simulink model "potential_field_controller"  (R2020b)
settings: Solver=VariableStepAuto  StartTime=0.0  StopTime=inf  RelTol=1e-3
values from neighbouring files (symbols this model uses):
  nObst = size(obstacles,2)    [setupPFC.m]
  obstacles = getObstaclepoints()    [setupPFC.m]
  timeDelay = FMS.Ts*4    [setupPFC.m]
  waypoints = getWaypoints()    [setupPFC.m]
undefined symbols (not defined in the file or in its folder): ssH, ssPitch, ssPitch2U, ssRoll, ssRoll2V, ssYaw
libraries: simulink x2, ARBlocks x1
settings Model: Creator=Adarsh  LastModifiedBy=Adarsh

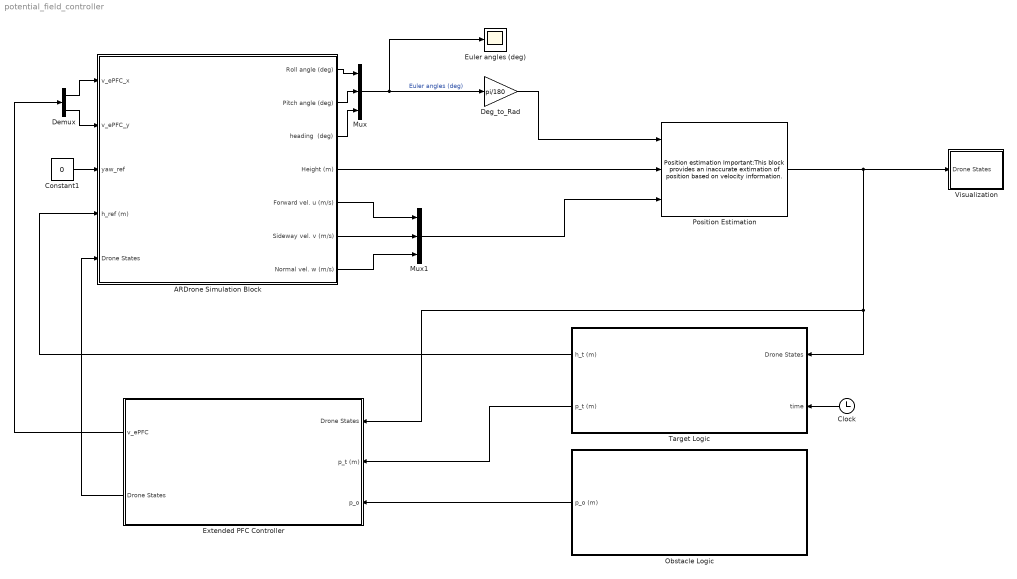
== system potential_field_controller ==
  ARDrone Simulation Block : Subsystem  AncestorBlock=ARBlocks/ARDrone Simulation Block
  Clock : Clock
  Constant1 : Constant  Value=0
  Deg_to_Rad : Gain  Gain=pi/180
  Demux : Demux  Outputs=2
  Euler angles (deg) : Scope
  Extended PFC Controller : Subsystem  AncestorBlock=ARBlocks/Baseline Controller
  Mux : Mux  Inputs=3
  Mux1 : Mux  Inputs=3
  Obstacle Logic : Subsystem  AncestorBlock=ARBlocks/Guidance logic
  "Position Estimation " : ARBlocks/Position estimation Important:This block provides an  inaccurate extimation of position  based on  velocity information.   SystemSampleTime=-1  VariantActivationTime=update diagram  Latency=0  AutoFrameSizeCalculation=off
  Target Logic : Subsystem  AncestorBlock=ARBlocks/Guidance logic
  Visualization : Subsystem
  wires:
  ARDrone Simulation Block/1(Roll angle (deg)) -> Mux/1
  ARDrone Simulation Block/2(Pitch angle (deg)) -> Mux/2
  ARDrone Simulation Block/3(heading  (deg)) -> Mux/3
  Deg_to_Rad/1 -> "Position Estimation "/1
  ARDrone Simulation Block/4(Height (m)) -> "Position Estimation "/2
  ARDrone Simulation Block/5(Forward vel. u (m/s)) -> Mux1/1
  ARDrone Simulation Block/6(Sideway vel. v (m/s)) -> Mux1/2
  ARDrone Simulation Block/7(Normal vel. w (m/s)) -> Mux1/3
  Mux1/1 -> "Position Estimation "/3
  "Position Estimation "/1 -> Visualization/1(Drone States), Target Logic/1(Drone States), Extended PFC Controller/1("Drone States ")
  Obstacle Logic/1(p_o (m)) -> Extended PFC Controller/3(p_o)
  Target Logic/2(p_t (m)) -> Extended PFC Controller/2(p_t (m))
  Target Logic/1(h_t (m)) -> ARDrone Simulation Block/4(h_ref (m))
  Clock/1 -> Target Logic/2(time)
  Mux/1 -> Euler angles (deg)/1, Deg_to_Rad/1  "Euler angles (deg)"
  Demux/1 -> ARDrone Simulation Block/1(v_ePFC_x)
  Demux/2 -> ARDrone Simulation Block/2(v_ePFC_y)
  Extended PFC Controller/1(v_ePFC) -> Demux/1
  Constant1/1 -> ARDrone Simulation Block/3(yaw_ref)
  Extended PFC Controller/2(Drone States) -> ARDrone Simulation Block/5(Drone States)

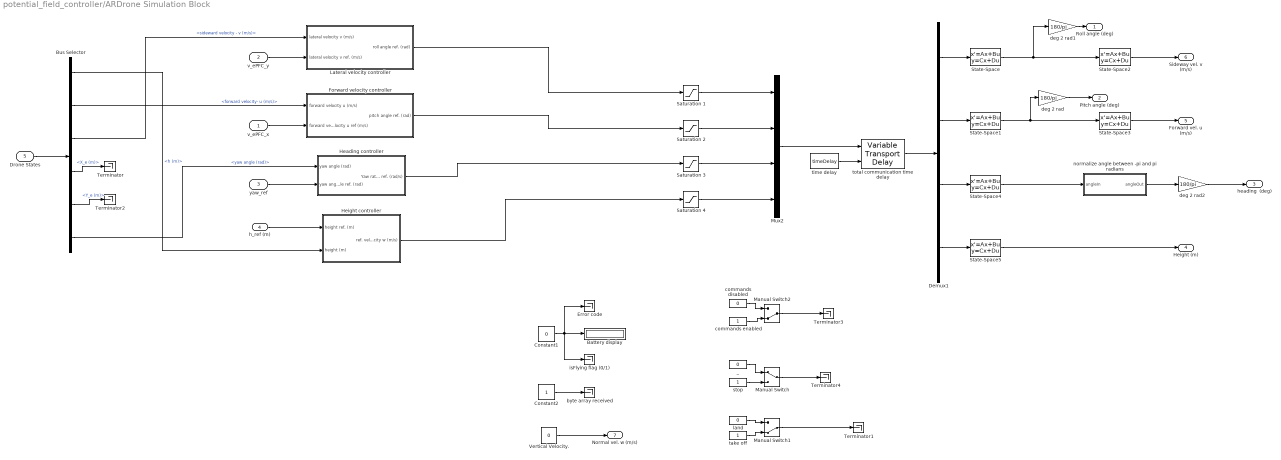
== system potential_field_controller/ARDrone Simulation Block ==
  v_ePFC_x : Inport
  v_ePFC_y : Inport  Port=2
  yaw_ref : Inport  Port=3
  h_ref (m) : Inport  Port=4
  Drone States : Inport  Port=5
  Battery display : Display
  Bus Selector : BusSelector  OutputSignals=h (m),forward velocity- u (m/s),sideward velocity - v (m/s),X_e (m),Y_e (m),yaw angle (rad)
  Constant1 : Constant  Value=0
  Constant2 : Constant
  Demux1 : Demux
  Error code : Terminator
  "Forward velocity controller " : Subsystem
  Heading controller : Subsystem
  "Height controller " : Subsystem
  Lateral velocity controller : Subsystem
  Manual Switch : ManualSwitch
  Manual Switch1 : ManualSwitch  CurrentSetting=0
  Manual Switch2 : ManualSwitch  CurrentSetting=0
  Mux2 : Mux
  Saturation {1..4} (4 alike) : Saturate  UpperLimit=1  LowerLimit=-1
  State-Space : StateSpace  A=ssRoll.a  B=ssRoll.b  C=ssRoll.c  D=ssRoll.d  InitialCondition=0
  State-Space1 : StateSpace  A=ssPitch.a  B=ssPitch.b  C=ssPitch.c  D=ssPitch.d  InitialCondition=0
  State-Space2 : StateSpace  A=ssRoll2V.a  B=ssRoll2V.b  C=ssRoll2V.c  D=ssRoll2V.d  InitialCondition=0
  State-Space3 : StateSpace  A=ssPitch2U.a  B=ssPitch2U.b  C=ssPitch2U.c  D=ssPitch2U.d  InitialCondition=0
  State-Space4 : StateSpace  A=ssYaw.a  B=ssYaw.b  C=ssYaw.c  D=ssYaw.d  InitialCondition=0
  State-Space5 : StateSpace  A=ssH.a  B=ssH.b  C=ssH.c  D=ssH.d  InitialCondition=0
  Terminator{,1..4} (5 alike) : Terminator
  "Vertical Velocity. " : Constant  Value=0
  _ : Constant  Value=0
  byte array received : Terminator
  commands disabled : Constant  Value=0
  commands enabled : Constant
  deg 2 rad : Gain  Gain=180/pi
  deg 2 rad1 : Gain  Gain=180/pi
  deg 2 rad2 : Gain  Gain=180/pi
  isFlying flag (0/1) : Terminator
  land : Constant  Value=0
  normalize angle between -pi and pi radians : MATLAB Function  TreatAsAtomicUnit=on
  stop : Constant
  take off : Constant
  time delay : Constant  Value=timeDelay
  total communication time delay : VariableTransportDelay  MaximumDelay=10  InitialOutput=[0 0 0 0]  MaximumPoints=4096
  Roll angle (deg) : Outport
  Pitch angle (deg) : Outport  Port=2
  heading  (deg) : Outport  Port=3
  Height (m) : Outport  Port=4
  Forward vel. u (m/s) : Outport  Port=5
  Sideway vel. v (m/s) : Outport  Port=6
  Normal vel. w (m/s) : Outport  Port=7
  wires:
  "Vertical Velocity. "/1 -> Normal vel. w (m/s)/1
  deg 2 rad2/1 -> heading  (deg)/1
  deg 2 rad1/1 -> Roll angle (deg)/1
  deg 2 rad/1 -> Pitch angle (deg)/1
  normalize angle between -pi and pi radians/1(angleOut) -> deg 2 rad2/1
  State-Space5/1 -> Height (m)/1
  State-Space3/1 -> Forward vel. u (m/s)/1
  State-Space2/1 -> Sideway vel. v (m/s)/1
  State-Space4/1 -> normalize angle between -pi and pi radians/1(angleIn)
  Demux1/3 -> State-Space4/1
  Demux1/2 -> State-Space1/1
  Saturation 4/1 -> Mux2/4
  Saturation 3/1 -> Mux2/3
  Saturation 2/1 -> Mux2/2
  Saturation 1/1 -> Mux2/1
  total communication time delay/1 -> Demux1/1
  Mux2/1 -> total communication time delay/1
  time delay/1 -> total communication time delay/2
  State-Space1/1 -> State-Space3/1, deg 2 rad/1
  State-Space/1 -> State-Space2/1, deg 2 rad1/1
  Demux1/4 -> State-Space5/1
  Demux1/1 -> State-Space/1
  "Height controller "/1(ref. velocity w (m/s)) -> Saturation 4/1
  "Forward velocity controller "/1(pitch angle ref. (rad)) -> Saturation 2/1
  Lateral velocity controller/1(roll angle ref. (rad)) -> Saturation 1/1
  land/1 -> Manual Switch1/1
  Manual Switch1/1 -> Terminator1/1
  take off/1 -> Manual Switch1/2
  commands disabled/1 -> Manual Switch2/1
  commands enabled/1 -> Manual Switch2/2
  Manual Switch2/1 -> Terminator3/1
  Manual Switch/1 -> Terminator4/1
  stop/1 -> Manual Switch/2
  _/1 -> Manual Switch/1
  Constant1/1 -> Battery display/1, Error code/1, isFlying flag (0/1)/1
  Constant2/1 -> byte array received/1
  yaw_ref/1 -> Heading controller/2(yaw angle ref. (rad))
  Heading controller/1(Yaw rate ref. (rad/s)) -> Saturation 3/1
  v_ePFC_y/1 -> Lateral velocity controller/2(lateral velocity v ref. (m/s))
  v_ePFC_x/1 -> "Forward velocity controller "/2(forward velocity u ref (m/s))
  h_ref (m)/1 -> "Height controller "/1(height ref. (m))
  Drone States/1 -> Bus Selector/1
  Bus Selector/1 -> "Height controller "/2(height (m))  "<h (m)>"
  Bus Selector/2 -> "Forward velocity controller "/1(forward velocity u (m/s))  "<forward velocity- u (m/s)>"
  Bus Selector/3 -> Lateral velocity controller/1(lateral velocity v (m/s))  "<sideward velocity - v (m/s)>"
  Bus Selector/6 -> Heading controller/1(yaw angle (rad))  "<yaw angle (rad)>"
  Bus Selector/4 -> Terminator/1  "<X_e (m)>"
  Bus Selector/5 -> Terminator2/1  "<Y_e (m)>"

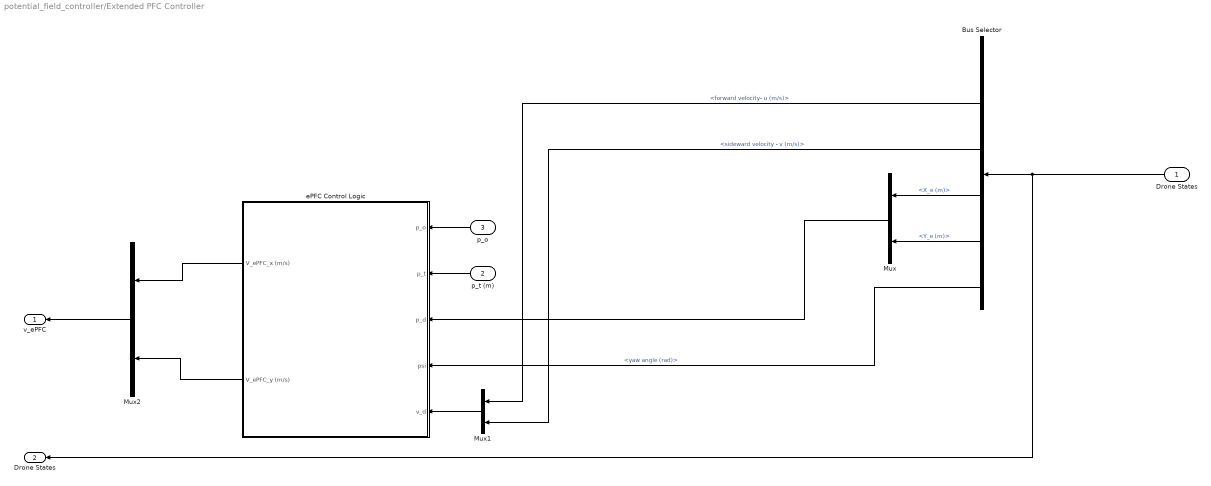
== system potential_field_controller/Extended PFC Controller ==
  "Drone States " : Inport
  p_t (m) : Inport  Port=2
  p_o : Inport  Port=3
  Bus Selector : BusSelector  OutputSignals=h (m),forward velocity- u (m/s),sideward velocity - v (m/s),X_e (m),Y_e (m),yaw angle (rad)
  Mux : Mux  Inputs=2
  Mux1 : Mux  Inputs=2
  Mux2 : Mux  Inputs=2
  ePFC Control Logic : Subsystem
  v_ePFC : Outport
  Drone States : Outport  Port=2
  wires:
  Bus Selector/6 -> ePFC Control Logic/4(psi)  "<yaw angle (rad)>"
  Bus Selector/2 -> Mux1/1  "<forward velocity- u (m/s)>"
  p_t (m)/1 -> ePFC Control Logic/2(p_t)
  Bus Selector/3 -> Mux1/2  "<sideward velocity - v (m/s)>"
  p_o/1 -> ePFC Control Logic/1(p_o)
  Bus Selector/4 -> Mux/1  "<X_e (m)>"
  Bus Selector/5 -> Mux/2  "<Y_e (m)>"
  Mux/1 -> ePFC Control Logic/3(p_d)
  Mux1/1 -> ePFC Control Logic/5(v_d)
  "Drone States "/1 -> Drone States/1, Bus Selector/1
  ePFC Control Logic/2(V_ePFC_y (m/s)) -> Mux2/2
  ePFC Control Logic/1(V_ePFC_x (m/s)) -> Mux2/1
  Mux2/1 -> v_ePFC/1

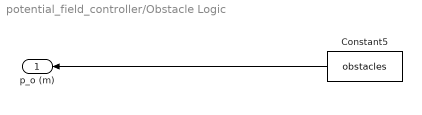
== system potential_field_controller/Obstacle Logic ==
  Constant5 : Constant  Value=obstacles  VectorParams1D=off
  p_o (m) : Outport
  wires:
  Constant5/1 -> p_o (m)/1

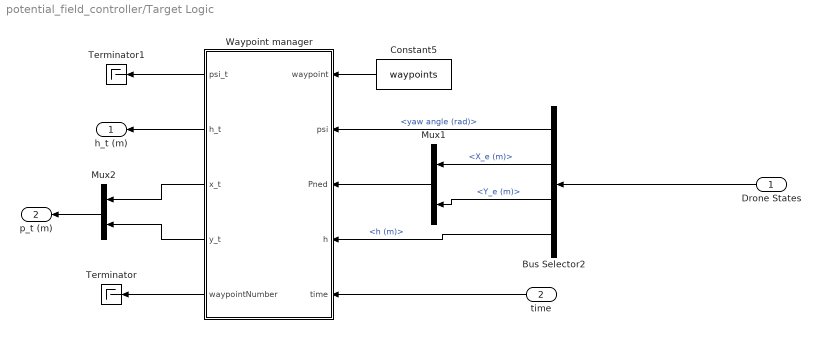
== system potential_field_controller/Target Logic ==
  Drone States : Inport
  time : Inport  Port=2
  Bus Selector2 : BusSelector  OutputSignals=yaw angle (rad),X_e (m),Y_e (m),h (m)
  Constant5 : Constant  Value=waypoints  VectorParams1D=off
  Mux1 : Mux  Inputs=2
  Mux2 : Mux  Inputs=2
  Terminator : Terminator
  Terminator1 : Terminator
  "Waypoint manager " : MATLAB Function  TreatAsAtomicUnit=on
  h_t (m) : Outport
  p_t (m) : Outport  Port=2
  wires:
  Constant5/1 -> "Waypoint manager "/1(waypoint)
  "Waypoint manager "/1(psi_t) -> Terminator1/1
  "Waypoint manager "/5(waypointNumber) -> Terminator/1
  Bus Selector2/4 -> "Waypoint manager "/4(h)  "<h (m)>"
  "Waypoint manager "/4(y_t) -> Mux2/2
  "Waypoint manager "/3(x_t) -> Mux2/1
  "Waypoint manager "/2(h_t) -> h_t (m)/1
  Mux1/1 -> "Waypoint manager "/3(Pned)
  Bus Selector2/1 -> "Waypoint manager "/2(psi)  "<yaw angle (rad)>"
  Bus Selector2/3 -> Mux1/2  "<Y_e (m)>"
  Bus Selector2/2 -> Mux1/1  "<X_e (m)>"
  Mux2/1 -> p_t (m)/1
  Drone States/1 -> Bus Selector2/1
  time/1 -> "Waypoint manager "/5(time)

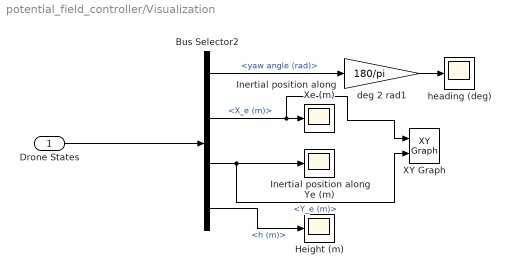
== system potential_field_controller/Visualization ==
  Drone States : Inport
  Bus Selector2 : BusSelector  OutputSignals=yaw angle (rad),X_e (m),Y_e (m),h (m)
  Height (m) : Scope
  Inertial position along Xe (m) : Scope
  Inertial position along Ye (m) : Scope
  XY Graph : simulink/Sinks/XY Graph  xmin=-3  xmax=3  ymin=-2  ymax=2  st=-1
  deg 2 rad1 : Gain  Gain=180/pi
  heading (deg) : Scope
  wires:
  Drone States/1 -> Bus Selector2/1
  Bus Selector2/1 -> deg 2 rad1/1  "<yaw angle (rad)>"
  Bus Selector2/2 -> XY Graph/1, Inertial position along Xe (m)/1  "<X_e (m)>"
  Bus Selector2/3 -> Inertial position along Ye (m)/1, XY Graph/2  "<Y_e (m)>"
  Bus Selector2/4 -> Height (m)/1  "<h (m)>"
  deg 2 rad1/1 -> heading (deg)/1

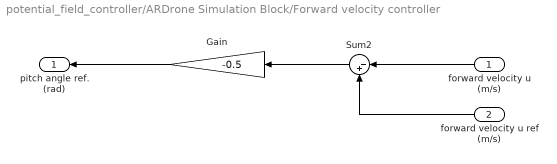
== system potential_field_controller/ARDrone Simulation Block/Forward velocity controller  ==
  forward velocity u (m/s) : Inport
  forward velocity u ref (m/s) : Inport  Port=2
  Gain : Gain  Gain=-0.5
  Sum2 : Sum  Inputs=|-+
  pitch angle ref. (rad) : Outport
  wires:
  forward velocity u (m/s)/1 -> Sum2/1
  Sum2/1 -> Gain/1
  Gain/1 -> pitch angle ref. (rad)/1
  forward velocity u ref (m/s)/1 -> Sum2/2

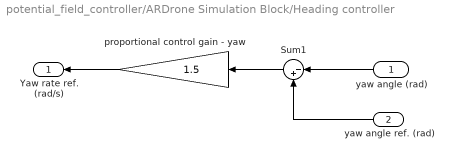
== system potential_field_controller/ARDrone Simulation Block/Heading controller ==
  yaw angle (rad) : Inport
  yaw angle ref. (rad) : Inport  Port=2
  Sum1 : Sum  Inputs=|-+
  proportional control gain - yaw : Gain  Gain=1.5
  Yaw rate ref. (rad/s) : Outport
  wires:
  yaw angle (rad)/1 -> Sum1/1
  proportional control gain - yaw/1 -> Yaw rate ref. (rad/s)/1
  Sum1/1 -> proportional control gain - yaw/1
  yaw angle ref. (rad)/1 -> Sum1/2

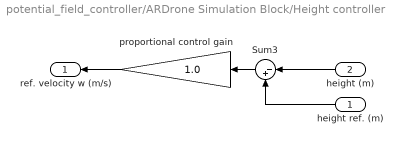
== system potential_field_controller/ARDrone Simulation Block/Height controller  ==
  height ref. (m) : Inport
  height (m) : Inport  Port=2
  Sum3 : Sum  Inputs=|-+
  proportional control gain : Gain  Gain=1.0
  ref. velocity w (m/s) : Outport
  wires:
  proportional control gain/1 -> ref. velocity w (m/s)/1
  Sum3/1 -> proportional control gain/1
  height (m)/1 -> Sum3/1
  height ref. (m)/1 -> Sum3/2

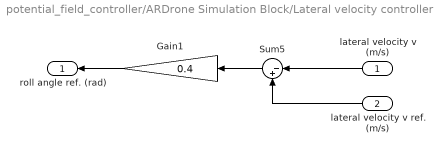
== system potential_field_controller/ARDrone Simulation Block/Lateral velocity controller ==
  lateral velocity v (m/s) : Inport
  lateral velocity v ref. (m/s) : Inport  Port=2
  Gain1 : Gain  Gain=0.4
  Sum5 : Sum  Inputs=|-+
  roll angle ref. (rad) : Outport
  wires:
  lateral velocity v (m/s)/1 -> Sum5/1
  Sum5/1 -> Gain1/1
  Gain1/1 -> roll angle ref. (rad)/1
  lateral velocity v ref. (m/s)/1 -> Sum5/2

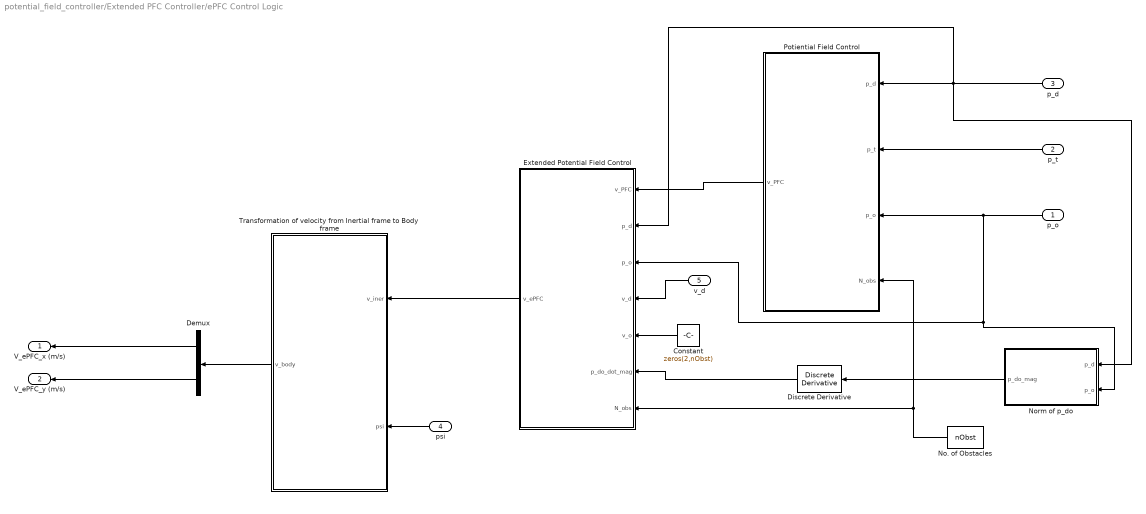
== system potential_field_controller/Extended PFC Controller/ePFC Control Logic ==
  p_o : Inport
  p_t : Inport  Port=2
  p_d : Inport  Port=3
  psi : Inport  Port=4
  v_d : Inport  Port=5
  Constant : Constant  Value=zeros(2,nObst)
  Demux : Demux  Outputs=2
  Discrete Derivative : simulink/Discrete/Discrete Derivative  gainval=1.0  ICPrevScaledInput=0.0  OutMin=[]  OutMax=[]  OutDataType=fixdt(1, 16)  OutScaling=2^-10  DoSatur=off
  Extended Potential Field Control : MATLAB Function  TreatAsAtomicUnit=on
  No. of Obstacles : Constant  Value=nObst  LockScale=on
  Norm of p_do : MATLAB Function  TreatAsAtomicUnit=on
  Potiential Field Control : MATLAB Function  TreatAsAtomicUnit=on
  "Transformation of velocity from Inertial frame to Body frame " : MATLAB Function  TreatAsAtomicUnit=on
  V_ePFC_x (m/s) : Outport
  V_ePFC_y (m/s) : Outport  Port=2
  wires:
  Demux/1 -> V_ePFC_x (m/s)/1
  "Transformation of velocity from Inertial frame to Body frame "/1(v_body) -> Demux/1
  Demux/2 -> V_ePFC_y (m/s)/1
  p_t/1 -> Potiential Field Control/2(p_t)
  p_o/1 -> Norm of p_do/2(p_o), Extended Potential Field Control/3(p_o), Potiential Field Control/3(p_o)
  psi/1 -> "Transformation of velocity from Inertial frame to Body frame "/2(psi)
  No. of Obstacles/1 -> Extended Potential Field Control/7(N_obs), Potiential Field Control/4(N_obs)
  p_d/1 -> Extended Potential Field Control/2(p_d), Potiential Field Control/1(p_d), Norm of p_do/1(p_d)
  v_d/1 -> Extended Potential Field Control/4(v_d)
  Potiential Field Control/1(v_PFC) -> Extended Potential Field Control/1(v_PFC)
  Discrete Derivative/1 -> Extended Potential Field Control/6(p_do_dot_mag)
  Extended Potential Field Control/1(v_ePFC) -> "Transformation of velocity from Inertial frame to Body frame "/1(v_iner)
  Norm of p_do/1(p_do_mag) -> Discrete Derivative/1
  Constant/1 -> Extended Potential Field Control/5(v_o)

== matlab function potential_field_controller/Extended PFC Controller/ePFC Control Logic/Potiential Field Control ==
  data: p_d input; p_t input; p_o input; v_PFC output; N_obs input
function v_PFC  = fcn(p_d , p_t, p_o, N_obs)
    %% Calculating PFC velocity
    % Inputs: drone position (X,Y), target positions (X,Y), 
    %         obstacle positions (X,Y), Number of Obstacles
    % Output: Computed PFC velocity in Inertial frame(m/s)
    
    p_avoid = 0.8; % Obstacle avoidance range (m)
       
    % Positive Scalar constants
    lamda_1 = 0.4; % Tuned values: 0.3 & 0.01
    eta_1 = 0.03;  
    
    v_att_PFC = -lamda_1 * (p_d - p_t); % attractive potential velocity
    v_rep_PFC = [0 ; 0]; % repulsive potential velocity
    
    for i = 1:N_obs
       if ((norm(p_d - p_o(:,i)) <= p_avoid) && (N_obs ~= 0))
            v_rep_PFC = v_rep_PFC + (eta_1/(norm(p_d-p_o(:,i)))^4) * (p_d - p_o(:,i)); 
       else 
            v_rep_PFC = v_rep_PFC + [0; 0]; 
       end
    end
    
    % Total PFC control velocity
    v_PFC = v_att_PFC + v_rep_PFC;
end

== matlab function potential_field_controller/Extended PFC Controller/ePFC Control Logic/Extended Potential Field Control ==
  data: v_PFC input; p_d input; p_o input; v_d input; v_o input; p_do_dot_mag input; v_ePFC output; N_obs input
function v_ePFC  = fcn(v_PFC, p_d , p_o, v_d, v_o, p_do_dot_mag, N_obs)    
    %% Calculating ePFC velocity
    % Inputs: PFC velocity (m/s), drone position (X,Y),  
    %         obstacle positions (X,Y), drone velocities (X,Y)
    %         obstacle velocities (X,Y), |p_do|_dot, No. of Obstacles
    % Output: Computed extended PFC velocity in Inertial frame (m/s)
    
    % Positive scalar constants
    lamda_2 = 0.3;
    eta_2 = 0.06; 
    eta_3 = 0.06; 
    
    v_att_ePFC = -lamda_2 * (v_d); % Here, v_target = 0
    v_rep1_ePFC = [0 ; 0];
    v_rep2_ePFC = [0 ; 0];
        
    for i = 1:N_obs
       if (((norm(v_o(:,i)) ~= 0)) && (N_obs ~= 0))
            v_rep1_ePFC = v_rep1_ePFC + (eta_2/(norm(v_d-v_o(:,i)))^4) * (v_d - v_o(:,i)); 
       else 
           v_rep1_ePFC = v_rep1_ePFC + [0;0]; % if v_obstacle = 0, no repulsive effect
       end
       
       if ((p_do_dot_mag(i) < 0) && (N_obs ~= 0))
           v_rep2_ePFC = v_rep2_ePFC + (eta_3 * p_do_dot_mag(i)) * ((p_d - p_o(:,i))/norm(p_d - p_o(:,i))); 
       else 
           v_rep2_ePFC = v_rep2_ePFC + [0;0]; % if |p_do_dot| >= 0, no repulsive effect
       end 
    end
    
    % Total ePFC control velocity
    v_ePFC = v_PFC + v_att_ePFC + v_rep1_ePFC - v_rep2_ePFC;
    
end

== matlab function potential_field_controller/Extended PFC Controller/ePFC Control Logic/Norm of p_do ==
  data: p_d input; p_do_mag output; p_o input; nObst parameter
function p_do_mag = fcn(p_d, p_o, nObst)
    
    p = zeros(1, nObst);
    
    if (nObst ~= 0)
        for i = 1:nObst
           p(i) = norm(p_d - p_o(:,i));
        end
    end
    
    p_do_mag = p;
    
end

== matlab function potential_field_controller/ARDrone Simulation Block/normalize angle between -pi and pi radians ==
  data: angleIn input; angleOut output
function angleOut = fcn(angleIn)
%#codegen

angleOut = mod(angleIn, 2*pi) ;
if angleOut > pi
    angleOut = -2*pi + angleOut ; 
end

== matlab function potential_field_controller/Extended PFC Controller/ePFC Control Logic/Transformation of velocity from Inertial frame to Body frame  ==
  data: v_iner input; v_body output; psi input
function v_body  = fcn(v_iner , psi)
    
    R = [cos(psi) sin(psi) ; -sin(psi) cos(psi)] ; 

    v_body = R * v_iner(1:2,1); 

end

== matlab function potential_field_controller/Target Logic/Waypoint manager  ==
  settings: updateMethod=DISCRETE
  data: psi_t output; h_t output; waypoint input; psi input; Pned input; h input; x_t output; y_t output; time input; waypointNumber output
function [psi_t, h_t,  x_t, y_t, waypointNumber]       = fcn(waypoint, psi, Pned, h, time )

    % Waypoint matrix contains final position, orientation, and waiting time.

    % Number of waypoints
    nPoints = size(waypoint, 2) ;

    % Persitent variable used to keep trak of next waypoint
    persistent wpointer;

    % Time zero for each waypoint. This is used to wait at a desired position.
    persistent t0 ;

    % Init. persistent variables
    if isempty(wpointer)
        wpointer = 1;
    end

    if isempty(t0)
        t0 = 0;
    end

    % A waypoint is reached if the distance between the desired waypoint and 
    % the vehicle is less than 0.1 m in the XY plane, less than 0.1 m in height, 
    % and less than 5 degrees in  heading. 

    if ( norm(Pned(1:2,1) - waypoint(1:2, wpointer) )< 0.1 && ...
            norm(h - waypoint(3, wpointer)) < 0.1  && norm(psi - waypoint(4, wpointer) )< 5*pi/180   )

        if(wpointer ~= nPoints)

            if (t0 ==0)
                t0 = time;
            else
                if (time - t0 > waypoint(5, wpointer))

                     if(wpointer < nPoints)
                        wpointer = wpointer+ 1;
                        t0 = 0;
                     end

                end
            end


        end



    end


    %% Outputs:
    h_t = waypoint(3, wpointer) ;
    psi_t = waypoint(4, wpointer) ;
    x_t = waypoint(1, wpointer) ;
    y_t = waypoint(2, wpointer) ;
    waypointNumber = wpointer ; 
end
